simulink model "lab4"  (R2024a)
settings: Solver=VariableStepAuto  StartTime=0.0  StopTime=100  RelTol=1e-3
settings Model: Creator=u5673749  LastModifiedBy=u5673749

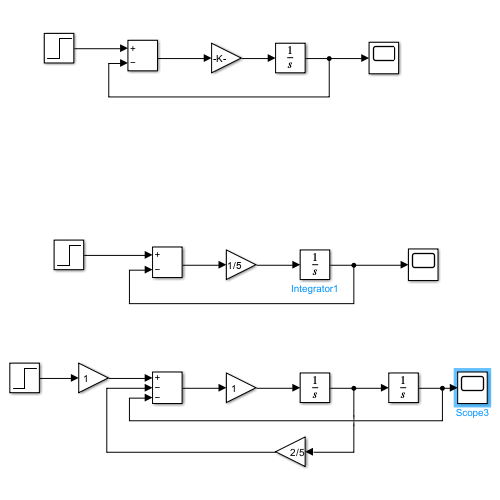
[thumbnail: Simulink's stored preview of the top-level diagram]
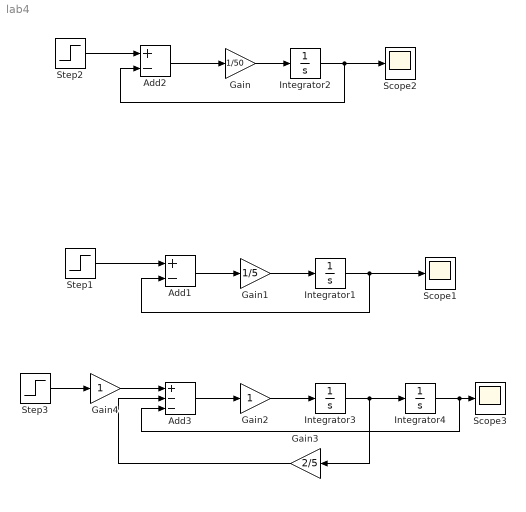
== system lab4 ==
  Add1 : Sum  Inputs=+-
  Add2 : Sum  Inputs=+-
  Add3 : Sum  Inputs=+--
  Gain : Gain  Gain=1/50
  Gain1 : Gain  Gain=1/5
  Gain2 : Gain
  Gain3 : Gain  Gain=2/5
  Gain4 : Gain
  Integrator{1..4} (4 alike) : Integrator
  Scope1 : Scope
  Scope2 : Scope
  Scope3 : Scope
  Step1 : Step  SampleTime=0
  Step2 : Step  Time=25  SampleTime=0
  Step3 : Step  SampleTime=0
  wires:
  Step1/1 -> Add1/1
  Add1/1 -> Gain1/1
  Gain1/1 -> Integrator1/1
  Integrator1/1 -> Scope1/1, Add1/2
  Step2/1 -> Add2/1
  Add2/1 -> Gain/1
  Gain/1 -> Integrator2/1
  Integrator2/1 -> Scope2/1, Add2/2
  Add3/1 -> Gain2/1
  Gain2/1 -> Integrator3/1
  Integrator3/1 -> Integrator4/1, Gain3/1
  Integrator4/1 -> Scope3/1, Add3/3
  Gain3/1 -> Add3/2
  Gain4/1 -> Add3/1
  Step3/1 -> Gain4/1
